simulink model "Path"  (R2016a)
settings: Solver=FixedStepAuto  StartTime=0.0  StopTime=50  FixedStep=0.01  RelTol=1e-3
settings Model: Creator=maximilian  LastModifiedBy=max
settings DataIOCC: SaveOutput=off  SaveTime=off

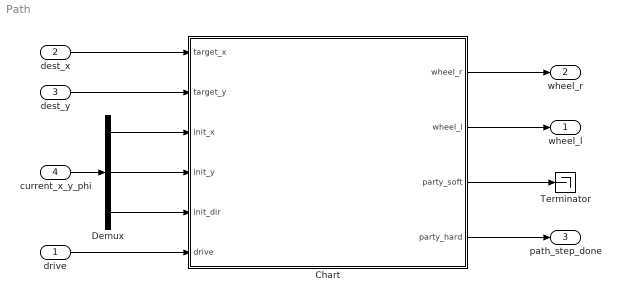
== system Path ==
  drive : Inport
  dest_x : Inport  Port=2
  dest_y : Inport  Port=3
  current_x_y_phi : Inport  Port=4
  Chart : Stateflow chart  TreatAsAtomicUnit=on
  Demux : Demux  Outputs=3
  Terminator : Terminator
  wheel_l : Outport
  wheel_r : Outport  Port=2
  path_step_done : Outport  Port=3
  wires:
  dest_x/1 -> Chart/1(target_x)
  dest_y/1 -> Chart/2(target_y)
  current_x_y_phi/1 -> Demux/1
  Demux/1 -> Chart/3(init_x)
  Demux/2 -> Chart/4(init_y)
  Demux/3 -> Chart/5(init_dir)
  Chart/4(party_hard) -> path_step_done/1
  Chart/2(wheel_l) -> wheel_l/1
  Chart/1(wheel_r) -> wheel_r/1
  Chart/3(party_soft) -> Terminator/1
  drive/1 -> Chart/6(drive)

== stateflow chart Path/Chart ==
  state compute
    entry:
    curr_x = init_x
    curr_y = init_y
    curr_dir = init_dir
    target_dir = atan2((target_y - curr_y), (target_x - curr_x))
    dir = (target_dir - curr_dir) / rad_per_sec
    dist = sqrt((target_y - curr_y)^2 + (target_x - curr_x)^2) / dist_per_sec
  state rotate_left
    entry:
    wheel_r = 1
    wheel_l = -1
  state rotate_right
    entry:
    wheel_r = -1
    wheel_l = 1
  state drive
    entry:
    party_soft = 1
    wheel_r = 1
    wheel_l = 1
  state profit
    entry:
    party_hard = 1
    wheel_l = 0
    wheel_r = 0
  (default) -> compute
  compute -> rotate_right [order 2] : [dir < 0]
  compute -> drive [order 3] : [dir == 0]
  compute -> rotate_left [order 1] : [dir > 0]
  rotate_right -> drive : [after(dir, sec)]
  rotate_left -> drive : [after(dir, sec)]
  drive -> profit : [after(dist, sec)]
  data: dist_per_sec constant double =0.1; target_x input; target_y input; init_x input; rad_per_sec constant double =0.1; wheel_r output; wheel_l output; target_dir local; curr_y local; curr_x local; dir local; curr_dir local; dist local; party_soft output; init_y input; init_dir input; party_hard output; drive input
